simulink library "uavsimBlockset_AugmentWind"  (Simulink 8.0)
settings: Solver=ode45  StartTime=0.0  StopTime=10.0  RelTol=1e-3
undefined symbols (not defined in the file): omegaw_bfrozen_rps, Vw_bfrozen_mps
settings Model: Creator=mstolle  LastModifiedBy=j.bolting

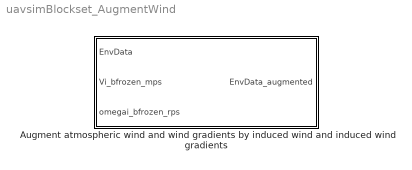
== system uavsimBlockset_AugmentWind ==
  Augment atmospheric wind and wind gradients by induced wind and induced wind gradients : Subsystem

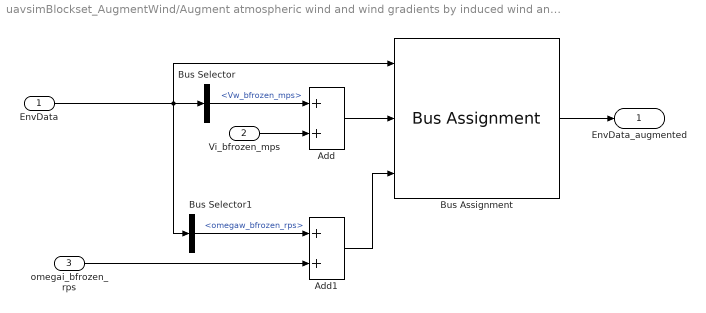
== system uavsimBlockset_AugmentWind/Augment atmospheric wind and wind gradients by induced wind and induced wind gradients ==
  EnvData : Inport  OutDataTypeStr=Bus: Environment
  Vi_bfrozen_mps : Inport  Port=2
  omegai_bfrozen_rps : Inport  Port=3
  Add : Sum
  Add1 : Sum
  Bus Assignment : BusAssignment  AssignedSignals=Vw_bfrozen_mps,omegaw_bfrozen_rps
  Bus Selector : BusSelector  OutputSignals=Vw_bfrozen_mps
  Bus Selector1 : BusSelector  OutputSignals=omegaw_bfrozen_rps
  EnvData_augmented : Outport  OutDataTypeStr=Bus: Environment
  wires:
  EnvData/1 -> Bus Selector1/1, Bus Selector/1, Bus Assignment/1
  Bus Selector/1 -> Add/1  "<Vw_bfrozen_mps>"
  Vi_bfrozen_mps/1 -> Add/2
  Add/1 -> Bus Assignment/2
  Bus Selector1/1 -> Add1/1  "<omegaw_bfrozen_rps>"
  omegai_bfrozen_rps/1 -> Add1/2
  Add1/1 -> Bus Assignment/3
  Bus Assignment/1 -> EnvData_augmented/1
